simulink model "NeuralNetworkSim"  (R2024a)
settings: Solver=FixedStepAuto  StartTime=0.0  StopTime=100000  RelTol=1e-3
undefined symbols (not defined in the file or in its folder): a_coeff, a_coeff_10, a_coeff_40, a_coeff_5, b_coeff, b_coeff_10, b_coeff_40
libraries: slpidlib x1
settings Model: Creator=kinsley  LastModifiedBy=kinsley

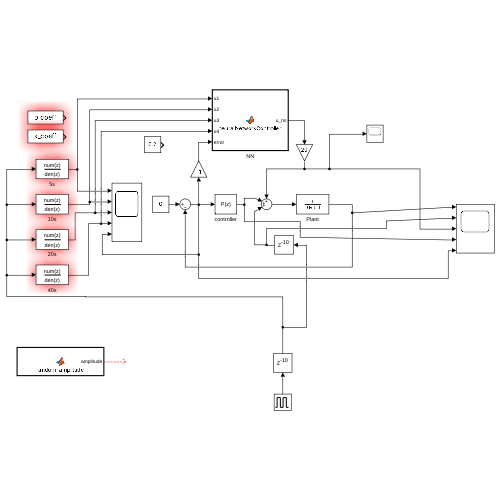
[thumbnail: Simulink's stored preview of the top-level diagram]
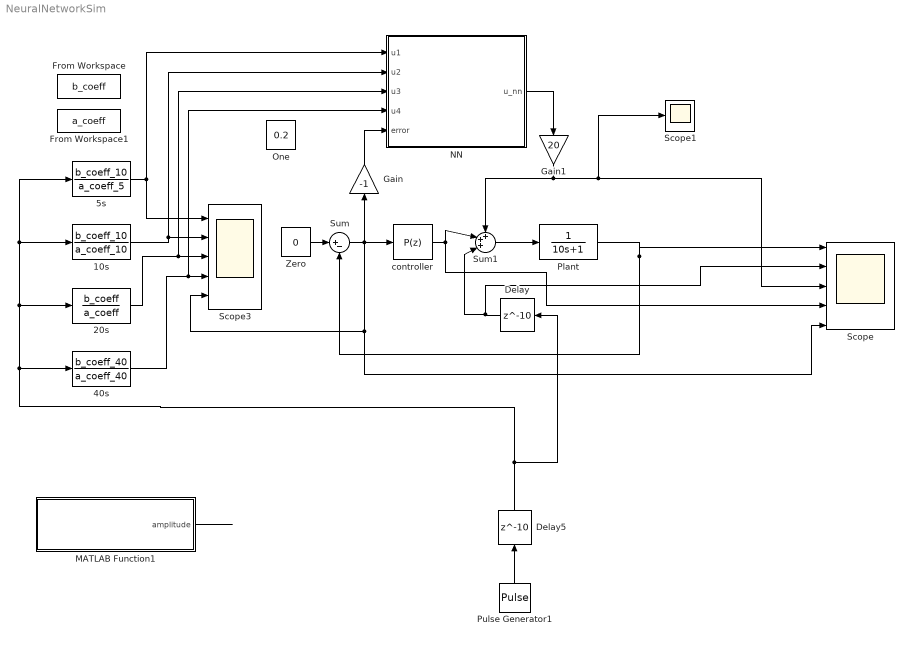
== system NeuralNetworkSim ==
  10s : DiscreteFilter  Numerator=b_coeff_10  Denominator=a_coeff_10
  20s : DiscreteFilter  Numerator=b_coeff  Denominator=a_coeff
  40s : DiscreteFilter  Numerator=b_coeff_40  Denominator=a_coeff_40
  5s : DiscreteFilter  Numerator=b_coeff_10  Denominator=a_coeff_5
  Delay : Delay  DelayLength=10
  Delay5 : Delay  DelayLength=10
  From Workspace : FromWorkspace  VariableName=b_coeff
  From Workspace1 : FromWorkspace  VariableName=a_coeff
  Gain : Gain  Gain=-1
  Gain1 : Gain  Gain=20
  MATLAB Function1 : MATLAB Function  TreatAsAtomicUnit=on
  NN : MATLAB Function  TreatAsAtomicUnit=on
  One : Constant  Value=0.2  OutDataTypeStr=Inherit: Inherit via back propagation
  Plant : TransferFcn  Denominator=[10 1]
  Pulse Generator1 : DiscretePulseGenerator  PulseType=Time based  Amplitude=0.3  Period=20  PulseWidth=2
  Scope : Scope  NumInputPorts=5
  Scope1 : Scope
  Scope3 : Scope  NumInputPorts=5
  Sum : Sum  Inputs=|+-
  Sum1 : Sum  Inputs=+++|
  Zero : Constant  Value=0  OutDataTypeStr=Inherit: Inherit via back propagation
  controller : slpidlib/PID Controller  Controller=P  Form=Parallel  TimeDomain=Discrete-time  UseExternalTs=off  SampleTime=-1  IntegratorMethod=Forward Euler  FilterMethod=Forward Euler  ControllerParametersSource=internal  P=20  I=1  UseKiTs=off  D=0  UseExternalDerivativeSource=off  N=100  UseFilter=on  TunerSelectOption=Transfer Function Based (PID Tuner App)  InitialConditionSource=internal  InitialConditionForIntegrator=0  InitialConditionForFilter=0  DifferentiatorICPrevScaledInput=0  ExternalReset=none  TrackingMode=off  Kt=1  LimitOutput=off  SatLimitsSource=internal  UpperSaturationLimit=inf  LowerSaturationLimit=-inf  LinearizeAsGain=on  AntiWindupMode=none  Kb=1  LimitIntegrator=off  UpperIntegratorSaturationLimit=inf  LowerIntegratorSaturationLimit=-inf  POutMin=[]  POutMax=[]  IOutMin=[]  IOutMax=[]  DOutMin=[]  DOutMax=[]  NOutMin=[]  NOutMax=[]  SumOutMin=[]  SumOutMax=[]  SaturationOutMin=[]  SaturationOutMax=[]  PParamMin=[]  PParamMax=[]  IParamMin=[]  IParamMax=[]  DParamMin=[]  DParamMax=[]  NParamMin=[]  NParamMax=[]  KbParamMin=[]  KbParamMax=[]  KtParamMin=[]  KtParamMax=[]  KbOutMin=[]  KbOutMax=[]  KtOutMin=[]  KtOutMax=[]  IntegratorOutMin=[]  IntegratorOutMax=[]  FilterOutMin=[]  FilterOutMax=[]  SumI1OutMin=[]  SumI1OutMax=[]  SumI2OutMin=[]  SumI2OutMax=[]  SumI3OutMin=[]  SumI3OutMax=[]  SumI4OutMin=[]  SumI4OutMax=[]  SumDOutMin=[]  SumDOutMax=[]  DifferentiatorOutMin=[]  DifferentiatorOutMax=[]  FilterDiffOutCoefMin=[]  FilterDiffOutCoefMax=[]  ReciprocalOutMin=[]  ReciprocalOutMax=[]  SumDenOutMin=[]  SumDenOutMax=[]  SumNumOutMin=[]  SumNumOutMax=[]  DivideOutMin=[]  DivideOutMax=[]  UdiffTsProdOutMin=[]  UdiffTsProdOutMax=[]  NTsProdOutMin=[]  NTsProdOutMax=[]  UintegralTsProdOutMin=[]  UintegralTsProdOutMax=[]  UngainTsProdOutMin=[]  UngainTsProdOutMax=[]  ClampingZeroOutDataTypeStr=Inherit: Inherit via back propagation  ClampingZeroOutMin=[]  ClampingZeroOutMax=[]  FilterDenConstantOutDataTypeStr=Inherit: Inherit via back propagation  FilterDenConstantOutMin=[]  FilterDenConstantOutMax=[]  PCopyOutDataTypeStr=Inherit: Inherit via back propagation  PCopyOutMin=[]  PCopyOutMax=[]  NCopyOutDataTypeStr=Inherit: Inherit via back propagation  NCopyOutMin=[]  NCopyOutMax=[]  IntegratorContinuousStateAttributes=''  IntegratorStateMustResolveToSignalObject=off  IntegratorRTWStateStorageClass=Auto  FilterContinuousStateAttributes=''  FilterStateMustResolveToSignalObject=off  FilterRTWStateStorageClass=Auto  ParallelPVariant=InternalParameters  IdealPVariant=Disabled  IVariant=Disabled  DVariant=Disabled  IntegratorVariant=Disabled  SatVariant=Disabled  AWVariant=Disabled  PCopyVariant=Disabled  TRVariant=Disabled  FdbkBlocksVariant=Forward  IdealPFdbkVariant=Disabled  SatFdbkVariant=Disabled  DerivativeFilterVariant=Disabled  NVariant=Disabled  NCopyVariant=Disabled_SignalSpec  FilterICVariant=Disabled  IntegratorICVariant=Disabled  ExternalResetVariant=Disabled  TRSumVariant=Passthrough  SumFdbkVariant=Disabled  SumVariant=Passthrough_P  TsampFilterVariant=InternalTs  TsampNgainVariant=Passthrough  TsampIntegralVariant=Disabled_SignalSpec  ExternalSaturationOutDataTypeStr=Inherit: Same as second input  DerivativeSourceVariant=Disabled
  wires:
  Zero/1 -> Sum/1
  Sum/1 -> Gain/1, Scope3/5, Scope/5, controller/1
  Sum1/1 -> Plant/1
  Plant/1 -> Sum/2, Scope/1
  Delay/1 -> Sum1/3, Scope/2
  MATLAB Function1/1(amplitude) -> ?
  controller/1 -> Scope/4, Sum1/2
  Pulse Generator1/1 -> Delay5/1
  NN/1(u_nn) -> Gain1/1
  5s/1 -> Scope3/1, NN/1(u1)
  20s/1 -> NN/3(u3), Scope3/3
  40s/1 -> NN/4(u4), Scope3/4
  Delay5/1 -> 40s/1, 20s/1, 5s/1, 10s/1, Delay/1
  Gain1/1 -> Sum1/1, Scope/3, Scope1/1
  10s/1 -> NN/2(u2), Scope3/2
  Gain/1 -> NN/5(error)

== matlab function NeuralNetworkSim/MATLAB Function1 ==
  data: amplitude output
function amplitude = random_amplitude()
% 生成-1到1之间的随机数
amplitude = 2*rand - 1;
end

== matlab function NeuralNetworkSim/NN ==
  settings: updateMethod=DISCRETE
  data: u1 input; u2 input; u3 input; u4 input; u_nn output; error input
function u_nn  = neuralNetworkController(u1, u2, u3, u4, error)
%#codegen

persistent nn;

if isempty(nn)
    layers = [4, 10, 20, 1];
    activationFunctions = {'tanh', 'tanh', 'tanh'};
    learningRate = 0.01;
    nn = NeuralNetwork(layers, activationFunctions, learningRate);
end

input = [u1; u2; u3; u4];


nn = nn.updateWeights(input, error);


% 前向传播
[u_nn, ~]= nn.forward(input);

% 更新权重
end
